simulink model "BiT_Template_V4"  (R2025a)
settings: Solver=FixedStepAuto  StartTime=0.0  StopTime=50  FixedStep=0.005  RelTol=1e-3
StopFcn:
  | user_confirmed = true;
  | disp('Gestoppt?!')
  | 
  | % stop(t);
  | % delete(t);
  | 
  | %% Switch to Config Mode
  | %Tc3_AI.sysManager.ActivateConfiguration();
  | %
  | % Tc3_AI.SwitchToConfig('local')
  | %
  | % %save Solution
  | % Tc3_AI.SaveSolution();
  | %
  | % %% Close Aktive VS Instance
  | % Tc3_AI.closeVsInstance();
values from neighbouring files (symbols this model uses):
  omega0 = interp1(u_bp, w_tab, u0, 'linear')    [Parameters.m]
  zdot0 = 0    [Parameters.m]
libraries: simulink x1, slpidlib x1
settings Model: SimulationMode=external  Creator=clemensm  LastModifiedBy=Lenard
settings OptimizationCC: LocalBlockOutputs=off
settings RTWCC: SystemTargetFile=TwinCatGrt.tlc  GenCodeOnly=on  GenerateMakefile=off  TemplateMakefile=tcgrt_msbuild.tmf  TargetLang=C++  Description=TwinCAT GRT Target
settings STFCustomTargetCC: SystemTargetFile=TwinCatGrt.tlc  TargetLangStandard=C++11 (ISO)  MultiwordLength=2048.0  DynamicStringBufferSize=256.0  ConcurrentExecutionCompliant=on  CombineOutputUpdateFcns=on  CodeInterfacePackaging=Reusable function  CPPClassGenCompliant=on  GRTInterface=off  GenerateAllocFcn=on  TcCom_ExecutionInfoParam=on  TcCom_OutputCreateSymbols=on  TcProject_CreateScopedEnums=Auto  TcProject_UseTmxExtension=Auto  TcProject_PublishTcOSARMv7A=off  TcProject_SignWithTwinCatCertificate=inherit default  TcCom_ExtendSignalResolution=on  TcProject_DrvProductVersion=$<DrvFileVersion>  TcProject_DataExchangeModulesVersion=$<ModuleGenerator:DataExchange:Version>  TcCom_ParametersCreateSymbols=on  TcProject_PublishTcRTx64=on  TcCom_CallerVerification=Default  TcProject_UseIntrinsics=on  TcCom_OutputReadOnly=on  TcProject_DrvFileVersion=$<VersionFromFile>  TcProject_VendorIcon=$<TE140x:Icon>  TcProject_LibCatPath=$<Project:Dir>\$<Project:Name>.libcat.xml  TcProject_GenerateStructDutsWithDefaultValues=Auto  TcCom_ExecutionSequence=UpdateBeforeOutputMapping  TcCom_ExtModeRtAllowForParameterChange=on  TcPlcFb_InitExceptionHandling=CallerExceptions  TcCom_Generate=on  TcCom_DWorkCreateSymbols=on  TcProject_StaticStlStringCapacity=Auto  TcCom_DataStoreReadOnly=off  TcCom_ResolveMaskedSubsystems=on  TcCom_OnlineChange=off  TcProject_UseCodeInfoExporter=on  TcPlcFb_MonitorExecutionTime=off  TcCom_OriginalIoBlockNames=off  TcPlcFb_Generate=off  TcCom_StepSizeAdaptation=RequireMatchingTaskCycleTime  TcProject_CppLanguageStandard=Default  TcPlcFb_ExtModeRtAllowExecutionCommands=off  TcProject_PublishTcOSARMv8A=off  TcProject_GeneratePlcLibrary=off  TcCom_MonitorExecutionTime=off  TcProject_PublishTcOSx64=off  TcProject_UseCodeDescriptor=on  TcProject_TmxInstall=on  TcProject_PublishParallel=on  TcCom_DWorkReadOnly=on  TcCom_BlockIoDataAccess=Internal DataArea  TcCom_AllowDataAreaForSharedData=off  TcCom_InputReadOnly=off  TcCom_UpdateExceptionHandling=CallerExceptions  TcProject_Generate=on  TcProject_ProductName=$<ModuleGenerator:ProductId> $<ModuleGenerator:Version:MAJOR.MINOR>  TcCom_BlockIoReadOnly=on  TcProject_PlcVarPrefixes=PVOID=p | BOOL=b | BOOL32=b | DATE=d | TIME_OF_DATE=td | TIME=t | LTIME=t | GUID=n  TcCom_AccessLockState=Auto  TcCom_ParametersReadOnly=off  TcPlcFb_ExtModeRtWaitForStart=off  TcProject_LowestCompatibleTcBuild=$<TwinCAT:Version:BUILD>  TcCom_ContStateReadOnly=on  TcProject_PublishPlatformtoolset=Auto  TcProject_GenerateVsSolution=No  TcCom_BlockDiagramExport=on  TcCom_TcComWrapperFb=off  TcCom_StrictAccessLock=on  TcProject_PreferIntOverLong=off  TcProject_CoderCppNamespace=coder  TcProject_Description=TwinCAT executable file, generated by TwinCAT $<ModuleGenerator:ProductId>  TcCom_ExecutionInfoOutput=off  TcProject_SignTwinCatCertName=MCI_2024_OEM.tccert  TcProject_EnableNewPlatforms=off  TcProject_Versioning=Versioned  TcCom_InputDataAccess=Input Destination DataArea  TcProject_VersionSrc=$<LatestTMFile>  TcPlcFb_ExtModeRtAllowForParameterChange=off  TcProject_MaxVisibleArrayElements=200U  TcCom_BlockIoCreateSymbols=on  TcProject_UseNativeBlockDiagramExport=off  TcProject_BuildSystem=Auto  TcProject_UseDataExchangeModules=off  TcProject_ClassFactoryName=$<Project:Name>  TcCom_DataStoreCreateSymbols=on  TcProject_UseDescriptorCodeType=on  TcProject_PublishTcUMx86=off  TcProject_CLanguageStandard=Default  TcCom_ModuleCaller=CyclicTask  TcProject_VendorName=TE140x Module Vendor  TcProject_UseStaticStlString=off  TcProject_PublishTcOSARMv7M=off  TcCom_ContStateDataAccess=Internal DataArea  TcCom_BlockDiagramDebugInfoExport=on  TcCom_InitExceptionHandling=CallerExceptions  TcProject_PublishTcRTx86=on  TcCom_BlockDiagramVariableAccess=AssignToParent  TcCom_Legacy_ModuleBuildInfoParam=on  TcPlcFb_OemLicenses=$<Project:OemLicenses>  TcCom_OutputDataAccess=Output Source DataArea  TcCom_OemLicenses=$<Project:OemLicenses>  TcCom_ExecuteModelCode=on  TcCom_ParametersInitValues=on  TcCom_TcComWrapperFbProperties=off  TcCom_GroupIcon=$<TE140x:Icon>  TcCom_TcComWrapperFbPropertyMonitoring=NoMonitoring  TcCom_OnlineChangeRestoreDataAreas=off  TcProject_InstallPlcLibrary=off  TcCom_ExtModeRtWaitForStart=off  TcCom_ContStateCreateSymbols=on  TcCom_DWorkDataAccess=Internal DataArea  TcProject_PublishTcUMx64=off  TcProject_BuildWithWdk=inherit default  TcCom_GroupName=TE140x|Simulink Modules  TcProject_Publish=on  TcCom_InputCreateSymbols=on  TcProject_IncrementVersion=Revision  TcCom_VariableSymbolMapping=Identical  TcProject_CreateUniqueEnumItemNames=off  TcProject_DeployRestart=off  TcProject_PublishConfiguration=Release  TcCom_ParametersDataAccess=Internal DataArea  TcProject_Verbosity=Normal  TcProject_ProjectDir=C:\TwinCAT\3.1\CustomConfig\Modules\Ctrl_only  TcProject_Copyright=Copyright $<VendorName> $<LocalDateTime:%Y>  TcCom_ExtModeRtAllowExecutionCommands=on  TcProject_PreferToolArchitectureX64=on  TcCom_InputInitValues=off  TcProject_LibraryCategories=$<VendorName>  TcCom_DataStoreDataAccess=None  TcCom_ModuleIcon=$<TE140x:Icon>  TcProject_ForceRebuildForPublish=off  TcCom_GroupDisplayName=$<GroupName>  TcCom_GlobalParamDefaultSharing=Define  TcPlcFb_UpdateExceptionHandling=CallerExceptions
settings GRTTargetCC: ExtMode=on  ExtModeMexFile=TcExtModeClient  MultiInstanceErrorCode=None  TargetLangStandard=C++11 (ISO)  ParMdlRefBuildCompliant=off  CompOptLevelCompliant=off  MatFileLogging=off  CodeInterfacePackaging=Reusable function  GenerateAllocFcn=on  UseToolchainInfoCompliant=off

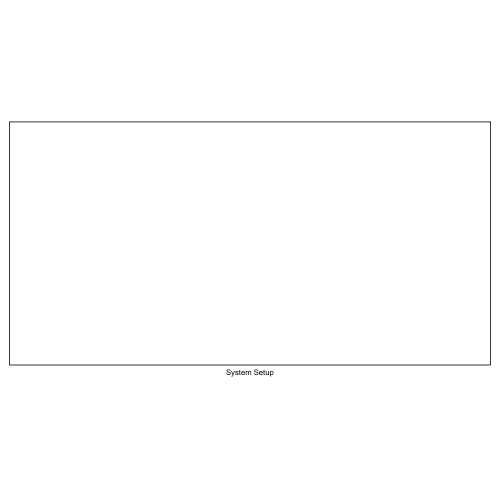
[thumbnail: Simulink's stored preview of the top-level diagram]
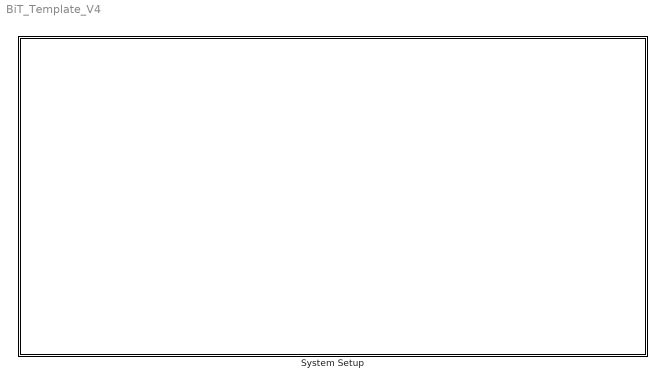
== system BiT_Template_V4 ==
  System Setup : Subsystem

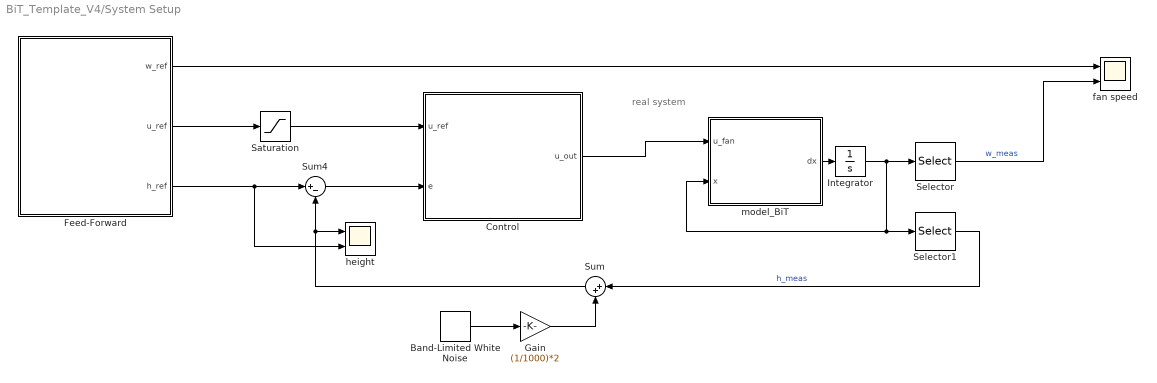
== system BiT_Template_V4/System Setup ==
  note: real system
  Band-Limited White Noise : simulink/Sources/Band-Limited White Noise  Cov=[0.1]  Ts=0.1  seed=[23341]
  Control : Subsystem
  Feed-Forward : Subsystem
  Gain : Gain  Gain=(1/1000)*2
  Integrator : Integrator  InitialCondition=[0.1;zdot0;omega0]  UpperSaturationLimit=0.35  LowerSaturationLimit=0
  Saturation : Saturate  UpperLimit=100  LowerLimit=0
  Selector : Selector  InputPortWidth=3  IndexOptions=Index vector (dialog)  Indices=3  OutputSizes=1
  Selector1 : Selector  InputPortWidth=3  IndexOptions=Index vector (dialog)  Indices=1  OutputSizes=1
  Sum : Sum  Inputs=|++
  Sum4 : Sum  Inputs=|+-
  fan speed : Scope  NumInputPorts=2
      settings: TimeSpan=60  ActiveDisplayYMinimum=4066.9032977047841  ActiveDisplayYMaximum=5105.1170189040668
  height : Scope  NumInputPorts=2
      settings: TimeSpan=60  ActiveDisplayYMinimum=-0.87290522466699971  ActiveDisplayYMaximum=1.7731695802829239  DataLoggingVariableName=ScopeData2
  model_BiT : MATLAB Function  TreatAsAtomicUnit=on
  wires:
  Selector/1 -> fan speed/2  "w_meas"
  model_BiT/1(dx) -> Integrator/1
  Integrator/1 -> Selector/1, Selector1/1, model_BiT/2(x)
  Feed-Forward/1(w_ref) -> fan speed/1
  Sum4/1 -> Control/2(e)
  Feed-Forward/2(u_ref) -> Saturation/1
  Feed-Forward/3(h_ref) -> height/2, Sum4/1
  Saturation/1 -> Control/1(u_ref)
  Selector1/1 -> Sum/1  "h_meas"
  Sum/1 -> Sum4/2, height/1
  Band-Limited White Noise/1 -> Gain/1
  Gain/1 -> Sum/2
  Control/1(u_out) -> model_BiT/1(u_fan)

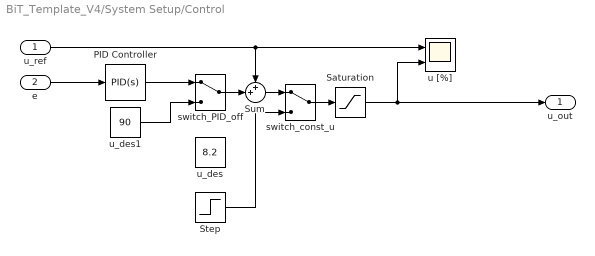
== system BiT_Template_V4/System Setup/Control ==
  u_ref : Inport
  e : Inport  Port=2
  PID Controller : slpidlib/PID Controller  Controller=PID  Form=Parallel  TimeDomain=Continuous-time  UseExternalTs=off  SampleTime=-1  IntegratorMethod=Forward Euler  FilterMethod=Forward Euler  ControllerParametersSource=internal  P=58.2445432756922  I=8.09148978156747  UseKiTs=off  D=79.7459625720082  UseExternalDerivativeSource=off  N=223.783259262105  UseFilter=on  TunerSelectOption=Transfer Function Based (PID Tuner App)  InitialConditionSource=internal  InitialConditionForIntegrator=0  InitialConditionForFilter=0  DifferentiatorICPrevScaledInput=0  ExternalReset=none  TrackingMode=off  Kt=1  LimitOutput=off  SatLimitsSource=internal  UpperSaturationLimit=inf  LowerSaturationLimit=-inf  LinearizeAsGain=on  AntiWindupMode=none  Kb=1  LimitIntegrator=off  UpperIntegratorSaturationLimit=inf  LowerIntegratorSaturationLimit=-inf  POutMin=[]  POutMax=[]  IOutMin=[]  IOutMax=[]  DOutMin=[]  DOutMax=[]  NOutMin=[]  NOutMax=[]  SumOutMin=[]  SumOutMax=[]  SaturationOutMin=[]  SaturationOutMax=[]  PParamMin=[]  PParamMax=[]  IParamMin=[]  IParamMax=[]  DParamMin=[]  DParamMax=[]  NParamMin=[]  NParamMax=[]  KbParamMin=[]  KbParamMax=[]  KtParamMin=[]  KtParamMax=[]  KbOutMin=[]  KbOutMax=[]  KtOutMin=[]  KtOutMax=[]  IntegratorOutMin=[]  IntegratorOutMax=[]  FilterOutMin=[]  FilterOutMax=[]  SumI1OutMin=[]  SumI1OutMax=[]  SumI2OutMin=[]  SumI2OutMax=[]  SumI3OutMin=[]  SumI3OutMax=[]  SumI4OutMin=[]  SumI4OutMax=[]  SumDOutMin=[]  SumDOutMax=[]  DifferentiatorOutMin=[]  DifferentiatorOutMax=[]  FilterDiffOutCoefMin=[]  FilterDiffOutCoefMax=[]  ReciprocalOutMin=[]  ReciprocalOutMax=[]  SumDenOutMin=[]  SumDenOutMax=[]  SumNumOutMin=[]  SumNumOutMax=[]  DivideOutMin=[]  DivideOutMax=[]  UdiffTsProdOutMin=[]  UdiffTsProdOutMax=[]  NTsProdOutMin=[]  NTsProdOutMax=[]  UintegralTsProdOutMin=[]  UintegralTsProdOutMax=[]  UngainTsProdOutMin=[]  UngainTsProdOutMax=[]  ClampingZeroOutDataTypeStr=Inherit: Inherit via back propagation  ClampingZeroOutMin=[]  ClampingZeroOutMax=[]  FilterDenConstantOutDataTypeStr=Inherit: Inherit via back propagation  FilterDenConstantOutMin=[]  FilterDenConstantOutMax=[]  PCopyOutDataTypeStr=Inherit: Inherit via back propagation  PCopyOutMin=[]  PCopyOutMax=[]  NCopyOutDataTypeStr=Inherit: Inherit via back propagation  NCopyOutMin=[]  NCopyOutMax=[]  IntegratorContinuousStateAttributes=''  IntegratorStateMustResolveToSignalObject=off  IntegratorRTWStateStorageClass=Auto  FilterContinuousStateAttributes=''  FilterStateMustResolveToSignalObject=off  FilterRTWStateStorageClass=Auto  ParallelPVariant=InternalParameters  IdealPVariant=Disabled  IVariant=InternalParameters  DVariant=InternalParameters  IntegratorVariant=Continuous  SatVariant=Disabled  AWVariant=Passthrough  PCopyVariant=Disabled  TRVariant=Disabled  FdbkBlocksVariant=Forward  IdealPFdbkVariant=Disabled  SatFdbkVariant=Disabled  DerivativeFilterVariant=ContFilter  NVariant=InternalParameters  NCopyVariant=Disabled  FilterICVariant=InternalICsFilter  IntegratorICVariant=InternalICs  ExternalResetVariant=Disabled  TRSumVariant=Passthrough  SumFdbkVariant=Disabled  SumVariant=Sum_PID  TsampFilterVariant=InternalTs  TsampNgainVariant=Passthrough  TsampIntegralVariant=Disabled_SignalSpec  ExternalSaturationOutDataTypeStr=Inherit: Same as second input  DerivativeSourceVariant=ErrorSignal  PreIntVariant=InternalPreInt
  Saturation : Saturate  UpperLimit=100  LowerLimit=0
  Step : Step  Time=30  Before=10  After=90  SampleTime=0.01
  Sum : Sum  Inputs=++|
  switch_PID_off : ManualSwitch
  switch_const_u : ManualSwitch
  u [%] : Scope  NumInputPorts=2
      settings: TimeSpan=60  ActiveDisplayYMinimum=2.4952441398406373  ActiveDisplayYMaximum=17.498295682149347
  u_des : Constant  Value=8.2
  u_des1 : Constant  Value=90
  u_out : Outport
  wires:
  e/1 -> PID Controller/1
  u_ref/1 -> u [%]/1, Sum/1
  Sum/1 -> switch_const_u/1
  PID Controller/1 -> switch_PID_off/1
  switch_PID_off/1 -> Sum/2
  u_des1/1 -> switch_PID_off/2
  Saturation/1 -> u_out/1, u [%]/2
  switch_const_u/1 -> Saturation/1
  Step/1 -> switch_const_u/2

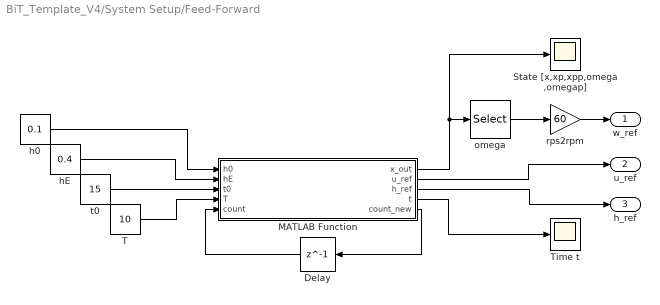
== system BiT_Template_V4/System Setup/Feed-Forward ==
  Delay : Delay  DelayLength=1
  MATLAB Function : MATLAB Function  TreatAsAtomicUnit=on
  State [x,xp,xpp,omega,omegap] : Scope
      settings: TimeSpan=60  ActiveDisplayYMinimum=-2.8507281834226665  ActiveDisplayYMaximum=4.5348179296068727
  T : Constant  Value=10
  Time t : Scope
      settings: ActiveDisplayYMinimum=-1  ActiveDisplayYMaximum=1
  h0 : Constant  Value=0.1
  hE : Constant  Value=0.4
  omega : Selector  InputPortWidth=5  IndexOptions=Index vector (dialog)  Indices=4  OutputSizes=1
  rps2rpm : Gain  Gain=60
  t0 : Constant  Value=15
  w_ref : Outport
  u_ref : Outport  Port=2
  h_ref : Outport  Port=3
  wires:
  h0/1 -> MATLAB Function/1(h0)
  omega/1 -> rps2rpm/1
  MATLAB Function/4(t) -> Time t/1
  T/1 -> MATLAB Function/4(T)
  t0/1 -> MATLAB Function/3(t0)
  Delay/1 -> MATLAB Function/5(count)
  MATLAB Function/5(count_new) -> Delay/1
  hE/1 -> MATLAB Function/2(hE)
  MATLAB Function/1(x_out) -> State [x,xp,xpp,omega,omegap]/1, omega/1
  MATLAB Function/2(u_ref) -> u_ref/1
  MATLAB Function/3(h_ref) -> h_ref/1
  rps2rpm/1 -> w_ref/1

== matlab function BiT_Template_V4/System Setup/model_BiT ==
  data: u_fan input; dx output; x input
function dx = model_BiT(u_fan, x)
%#codegen
% Plant "Ball in Tube" mit realer Lüfterkennlinie:
%   u_fan  : Duty in %
%   x      : [z; zdot; w]  (w in rpm)
%   dx     : [zdot; zddot; wdot]

% --- Parameter 
% Lüfter-Dynamik
% tau_omega = 1.4;                 % [s] Zeitkonstante PT1
tau_omega = 1.7217;
%k_omega = 39.125;

% Statische Kennlinie (Messpunkte)  u[%] -> w[rpm]
% -> 0% = 4000 rpm (Leerlauf), 10% = 4570 rpm, 90% = 7700 rpm
% u_bp  = [0    10    90    100];  % [%]
u_bp  = [0 2 5 8 10 12];  % [%]
% w_tab = [4000 4570  7700  7700]; % [rpm]
w_tab = [2950 3300 3650 4050 4250 4500]; % [rpm]

% Ball-/Rohr-Parameter
% a1 = 7.08e-4;
a1 = 7.4574e-04;
% a2 = 1.11;
a2 = 0.2237;
% a3 = 9.81;
a3 = 9.8100;

% Zustände 
z    = x(1);     % [m]
zdot = x(2);     % [m/s]
w    = x(3);     % [rpm]

% Balldynamik
zddot = (a1*w - a2*zdot)^2 - a3;

% --- Lüfter: statische Kennlinie + PT1-Dynamik 
% Eingangsgrenzen (SIM: 0..100 %; für reale HW ggf. 10..90 %)
u = max(0, min(100, u_fan));                     % clamp 0..100 %

% Statischer Sollwert der Drehzahl aus LUT
% (linear; bei Bedarf 'pchip' für glattere Kurve)
w_ss = interp1(u_bp, w_tab, u, 'linear', 'extrap');

% PT1 auf den statischen Sollwert
wdot = (w_ss - w) / tau_omega;                   % [rpm/s]
%wdot = (k_omega*(u_fan) - w)/tau_omega;

% --- Ausgabe 
dx = [zdot; zddot; wdot];
end

== matlab function BiT_Template_V4/System Setup/Feed-Forward/MATLAB Function ==
  data: x_out output; u_ref output; h0 input; hE input; t0 input; T input; h_ref output; t output; count input; count_new output
function [x_out, u_ref, h_ref, t, count_new] = feed_forward(h0, hE, t0, T, count)
% S-Kurven-Trajektorie + dynamische Vorsteuerung für den Lüfter
% Einheiten:
%   w in rpm, u_ref in % Duty, h in m (optional)
%
% Ein-/Ausgänge:
%   h0,hE  : Start/Ende der Höhe (nur Referenzanzeige, optional)
%   t0,T   : Startzeit-Offset, Trajektoriendauer
%   count  : Schrittzähler (diskret, aus deiner Sim)
%   u_ref  : Vorsteuerung in % Duty (an Summierstelle zum PID)
%   x_out  : [h_ref, dh/dt, d2h/dt2, w_ref[rps], wdot_ref[rps/s]]'
%
% 

% ===== Zeitbasis =====
dT = 0.005;                      
count_new = count + 1;
t = count_new*dT - t0;

% Ball-/Rohr-Parameter aus PT1 analyse
a1 = 7.08e-4;
a2 = 1.11;
a3 = 9.81;

% Lüfter Parameter 
tau = 1.4;                       % [s] Zeitkonstante PT1 (aus Messung)
k_omega = 39.125;                % [rpm/%] K Wert PT1 (aus Messung)
omega_bar = sqrt(a3)/a1;         % [rpm] Lüfterdrehzahl Arbeitspunkt

% Parameter aus linearisiertem State Space Model
alpha = 2*a1*a2*omega_bar;
beta  = 2*a1^2*omega_bar;
k     = k_omega;

% S-Kurve (quintic) für y=z (aus Lunze Kapitel 7.5)
if t <= 0
    r=0; s=0; ds=0; d2s=0; d3s=0;
elseif t >= T
    r=1; s=1; ds=0; d2s=0; d3s=0;
else
    r   = t / max(T,eps);
    s   = 10*r^3 - 15*r^4 + 6*r^5;
    ds  = (30*r.^2 - 60*r.^3 + 30*r.^4) / T;
    d2s = (60*r   - 180*r.^2 + 120*r.^3) / (T^2);
    d3s = (60     - 360*r    + 360*r.^2) / (T^3);
end

% Referenzhöhe und Ableitungen 
dz     = hE - h0;
h_ref  = h0 + dz*s;        % y_ref(t)  [m]
xp_ref = dz*ds;            % y'(t)     [m/s]
xpp_ref= dz*d2s;           % y''(t)    [m/s^2]
xppp_ref = dz*d3s;           % y'''(t)   [m/s^3]


% Vorsteuerung u_ff (inkrementell, um den AP) (aus Lunze Kapitel 7.5)
u_ff = (tau*xppp_ref + (tau*alpha + 1)*xpp_ref + alpha*xp_ref) / (beta*k);  % [%]

% Bias-Duty, damit Plant sofort "schwebt" 
u_eq = 7.5;                             % [%] (aus Kennlinie inverse LUT)
u_ref = min(max(u_eq + u_ff, 0), 100);  % absoluter Duty

% Omega (absolut) und Omega_dot (absolut) 
omega_tilde_rpm    = (xpp_ref + alpha*xp_ref) / beta;                 % [rpm] um Arbeitspunkt
omega_ref_rpm      = omega_bar + omega_tilde_rpm;                     % [rpm] mit Offset bei 0% dutycycle
omega_dot_tilde_rpm= (k/tau)*u_ff - (1/tau)*omega_tilde_rpm;          % [rpm/s] mit Offset bei 0% dutycycle

% Umwandlung in rps
omega_ref_rps      = omega_ref_rpm / 60;
omega_dot_ref_rps  = omega_dot_tilde_rpm / 60;

x_out = [h_ref, xp_ref, xpp_ref, omega_ref_rps, omega_dot_ref_rps]';
end
